simulink model "linear"  (R2016a)
settings: Solver=VariableStepAuto  StartTime=0.0  StopTime=10.0  RelTol=1e-3
undefined symbols (not defined in the file): DiscIntNeverNeededParam
libraries: aausat3_lib x1
settings Model: Creator=jn  LastModifiedBy=jn
settings DataIOCC: SaveFormat=Array
settings DebuggingCC: SolverPrmCheckMsg=warning  AllowSymbolicDim=off
settings ModelReferenceCC: PropagateSignalLabelsOutOfModel=off
settings ConfigComp: CovModelRefEnable=Off  CovSFcnEnable=off

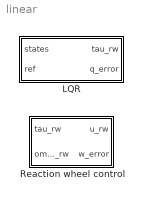
== system linear ==
  LQR : Subsystem
  Reaction wheel control : Subsystem  mask{omega_bias=0, Kp=0.02, Ki=0.06, Ts=0.1, u_bias=3.3/2}
      mask prompts: omega_bias "Bias angular velocity"; Kp "Motor Gain"; Ki "Integral gain"; Ts "Sampling time [s]"; u_bias "Bias voltage"

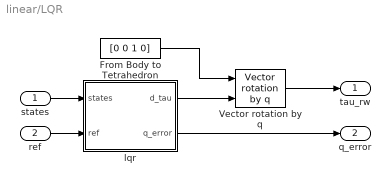
== system linear/LQR ==
  states : Inport  PortDimensions=[7 1]
  ref : Inport  Port=2  PortDimensions=[10 1]
  From Body to Tetrahedron : Constant  Value=[0 0 1 0]  VectorParams1D=off
  Vector rotation by q : aausat3_lib/Math Utilities/Quaternion operations/Vector rotation by q
  lqr : MATLAB Function  TreatAsAtomicUnit=on  SystemSampleTime=1
  tau_rw : Outport
  q_error : Outport  Port=2
  wires:
  ref/1 -> lqr/2(ref)
  states/1 -> lqr/1(states)
  lqr/2(q_error) -> q_error/1
  Vector rotation by q/1 -> tau_rw/1
  lqr/1(d_tau) -> Vector rotation by q/2
  From Body to Tetrahedron/1 -> Vector rotation by q/1

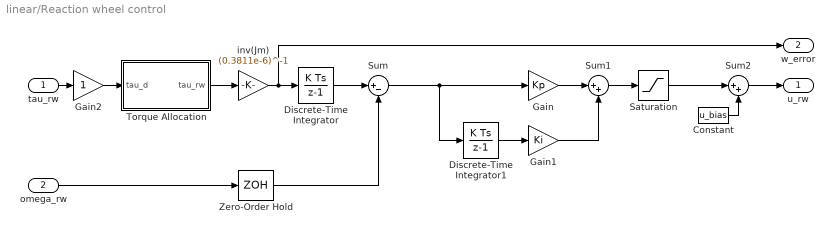
== system linear/Reaction wheel control ==
  tau_rw : Inport
  omega_rw : Inport  Port=2
  Constant : Constant  Value=u_bias
  Discrete-Time Integrator : DiscreteIntegrator  InitialCondition=omega_bias  InitialConditionSetting=State (most efficient)  LimitOutput=on  UpperSaturationLimit=1600  LowerSaturationLimit=0  ICPrevOutput=DiscIntNeverNeededParam  ICPrevScaledInput=DiscIntNeverNeededParam
  Discrete-Time Integrator1 : DiscreteIntegrator  InitialConditionSetting=State (most efficient)  SampleTime=Ts  LimitOutput=on  UpperSaturationLimit=100  LowerSaturationLimit=-100  ICPrevOutput=DiscIntNeverNeededParam  ICPrevScaledInput=DiscIntNeverNeededParam
  Gain : Gain  Gain=Kp
  Gain1 : Gain  Gain=Ki
  Gain2 : Gain
  Saturation : Saturate  UpperLimit=ones(4,1)*3.3/2  LowerLimit=-ones(4,1)*3.3/2
  Sum : Sum  Inputs=|+-
  Sum1 : Sum  Inputs=|++
  Sum2 : Sum  Inputs=|++
  Torque Allocation : MATLAB Function  TreatAsAtomicUnit=on
  Zero-Order Hold : ZeroOrderHold  SampleTime=Ts
  inv(Jm) : Gain  Gain=(0.3811e-6)^-1
  u_rw : Outport
  w_error : Outport  Port=2
  wires:
  inv(Jm)/1 -> w_error/1, Discrete-Time Integrator/1
  Discrete-Time Integrator/1 -> Sum/1
  omega_rw/1 -> Zero-Order Hold/1
  Torque Allocation/1(tau_rw) -> inv(Jm)/1
  Discrete-Time Integrator1/1 -> Gain1/1
  Gain/1 -> Sum1/1
  Gain1/1 -> Sum1/2
  Zero-Order Hold/1 -> Sum/2
  Sum1/1 -> Saturation/1
  Constant/1 -> Sum2/2
  Sum2/1 -> u_rw/1
  tau_rw/1 -> Gain2/1
  Gain2/1 -> Torque Allocation/1(tau_d)
  Saturation/1 -> Sum2/1
  Sum/1 -> Discrete-Time Integrator1/1, Gain/1

== matlab function linear/LQR/lqr ==
  data: states input; d_tau output; ref input; q_error output
function [d_tau,q_error] = fcn(states,ref)
%#codegen
q_i_s = states(1:4);
omega = states(5:7);
q_i_ref = ref(1:4);
omega_ref = ref(5:7);

q_i_s = qunit(q_i_s);
q_s_e = -qmult(q_i_ref,qinv(q_i_s));

x = [q_s_e(1:3); omega];
r = [[0 0 0]'; omega_ref];

K = [-0.3764    0.0116   -0.0046   -0.9056   -0.0000    0.0000
   -0.0120   -0.3945   -0.0173    0.0000   -0.9501    0.0000
    0.0055    0.0176   -0.4072    0.0000   -0.0000   -0.9803]*1.0e-3;

d_tau = K*(r-x);
q_error = q_s_e;

== matlab function linear/Reaction wheel control/Torque Allocation ==
  data: tau_d input; tau_rw output
function tau_rw = fcn(tau_d)
%#codegen
alpha = deg2rad(60);
beta = deg2rad(19.47);

P_w_th = [cos(beta)    -cos(beta)*cos(alpha)  -cos(beta)*cos(alpha)    0;
    0            cos(beta)*cos(alpha/2) -cos(beta)*cos(alpha/2)  0;
    -sin(beta)   -sin(beta)             -sin(beta)               1];

P_th_w = P_w_th'*(P_w_th*P_w_th')^-1;
tau_rw = P_th_w*tau_d;
